simulink model "TrafficLight"  (R2024b)
settings: Solver=VariableStepAuto  StartTime=0.0  StopTime=inf  RelTol=1e-3
settings Model: Creator=sudee  LastModifiedBy=sudee

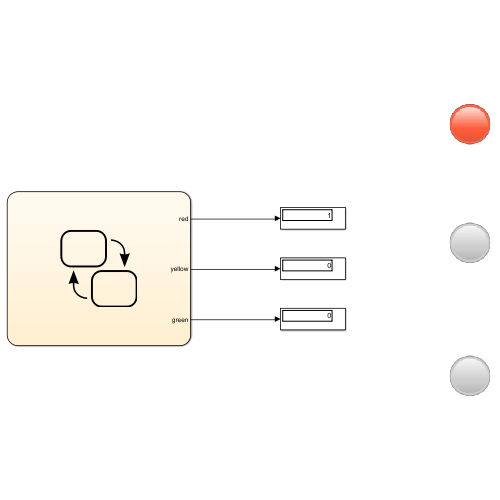
[thumbnail: Simulink's stored preview of the top-level diagram]
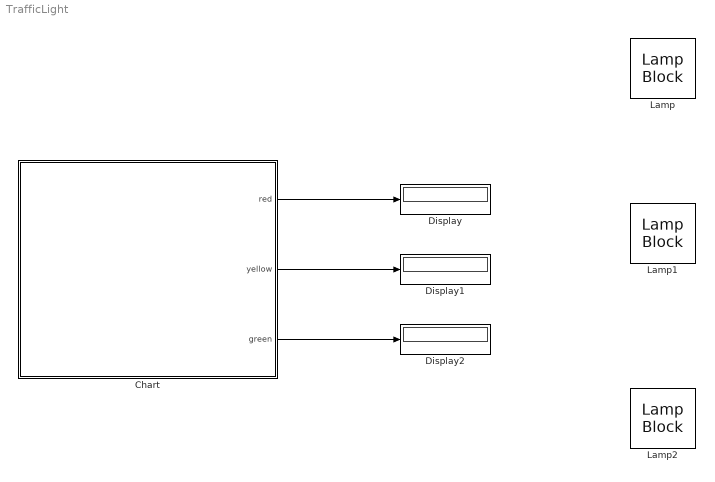
== system TrafficLight ==
  Chart : Stateflow chart  TreatAsAtomicUnit=on
  Display : Display
  Display1 : Display
  Display2 : Display
  Lamp : LampBlock  LabelPosition=Hide
  Lamp1 : LampBlock  LabelPosition=Hide
  Lamp2 : LampBlock  LabelPosition=Hide
  wires:
  Chart/3(green) -> Display2/1
  Chart/2(yellow) -> Display1/1
  Chart/1(red) -> Display/1

== stateflow chart TrafficLight/Chart ==
  state Go
    entry:
    yellow=0;
    during:
    green=1;
  state Be_Ready
    entry:
    red=0;
    during:
    yellow=1;
  state Stop
    entry:
    green=0;
    during:
    red=1;
  (default) -> Stop
  Be_Ready -> Go : [after(5, sec)]
  Stop -> Be_Ready : [after(5, sec)]
  Go -> Stop : [after(5, sec)]
  data: red output; yellow output; green output
